simulink model "crane"  (Simulink 7.0)
settings: Solver=ode3  StartTime=0.0  StopTime=T  FixedStep=stepsim  RelTol=1e-3
values from neighbouring files (symbols this model uses):
  A = [0 1 0 0;0 0 0 0;0 0 0 1;0 0 -eps(i)*g 0]    [EnsembleControlCrane.m]    (also in ThreePhaseEnsembleControlCrane.m; TwoPhaseEnsembleControlCrane.m)
  B = [0;1;0;-eps(i)]    [EnsembleControlCrane.m]    (also in ThreePhaseEnsembleControlCrane.m; TwoPhaseEnsembleControlCrane.m)
  C = eye([4 4])    [EnsembleControlCrane.m]    (also in ThreePhaseEnsembleControlCrane.m; TwoPhaseEnsembleControlCrane.m)
  D = [0;0;0;0]    [EnsembleControlCrane.m]    (also in ThreePhaseEnsembleControlCrane.m; TwoPhaseEnsembleControlCrane.m)
  start = [x_start,dxdt_start,theta,dthetadt_start]    [EnsembleControlCrane.m]    (also in ThreePhaseEnsembleControlCrane.m; TwoPhaseEnsembleControlCrane.m)
settings Model: Creator=Nathan  LastModifiedBy=Nathan

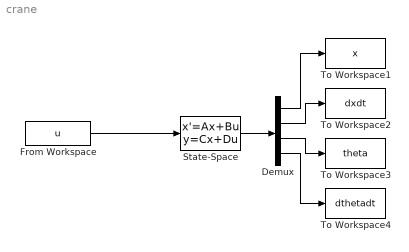
== system crane ==
  Demux : Demux
  From Workspace : FromWorkspace  VariableName=u  SampleTime=0
  State-Space : StateSpace  A=A  B=B  C=C  D=D  X0=start
  To Workspace1 : ToWorkspace  VariableName=x  SampleTime=-1  SaveFormat=Structure
  To Workspace2 : ToWorkspace  VariableName=dxdt  SampleTime=-1  SaveFormat=Structure
  To Workspace3 : ToWorkspace  VariableName=theta  SampleTime=-1  SaveFormat=Structure
  To Workspace4 : ToWorkspace  VariableName=dthetadt  SampleTime=-1  SaveFormat=Structure
  wires:
  From Workspace/1 -> State-Space/1
  State-Space/1 -> Demux/1
  Demux/1 -> To Workspace1/1
  Demux/2 -> To Workspace2/1
  Demux/3 -> To Workspace3/1
  Demux/4 -> To Workspace4/1
